simulink model "rccircuit"  (R2018b)
settings: Solver=VariableStepAuto  StartTime=0.0  StopTime=1  RelTol=1e-3
model workspace (MAT data in the model file):
  l = Simulink.Parameter
  l.Value = 10
  l.DataType = 'auto'
  l.Dimensions = [1 1]
  r = Simulink.Parameter
  r.Value = 750
  r.DataType = 'auto'
  r.Dimensions = [1 1]
  v = Simulink.Parameter
  v.Value = 5
  v.DataType = 'auto'
  v.Dimensions = [1 1]
settings Model: Creator=waleed.elbadry  LastModifiedBy=waleed.elbadry

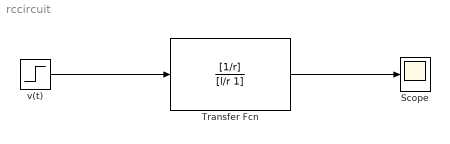
== system rccircuit ==
  Scope : Scope
  Transfer Fcn : TransferFcn  Numerator=[1/r]  Denominator=[l/r 1]
  v(t) : Step  Time=0  After=5  SampleTime=0
  wires:
  v(t)/1 -> Transfer Fcn/1
  Transfer Fcn/1 -> Scope/1
